simulink library "IO"  (R2024a)
settings: Solver=VariableStepAuto  StartTime=0.0  StopTime=10.0  RelTol=1e-3
values from neighbouring files (symbols this model uses):
  ADCBits = 12.0    [IO.sldd]
  DigitalPolarity : value not decoded    [IO.sldd]
  Vref = 5.0    [IO.sldd]
undefined symbols (not defined in the file or in its folder): Bridge, dt, enum2Raptor, H, raptor_xcp_function
libraries: Raptor_lib x118, Utilities x27, Cooling x1
(part 1 of 4)
settings Model: Creator=serga  LastModifiedBy=serga

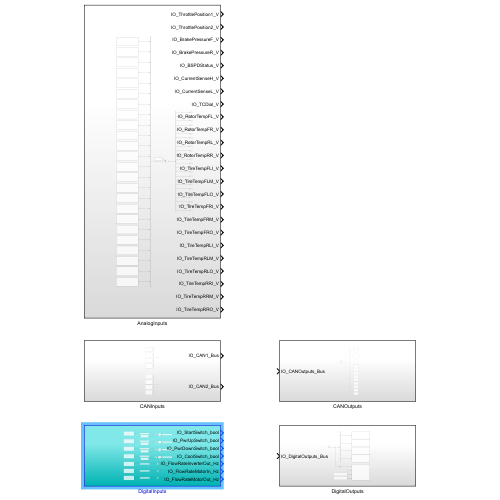
[thumbnail: Simulink's stored preview of the top-level diagram]
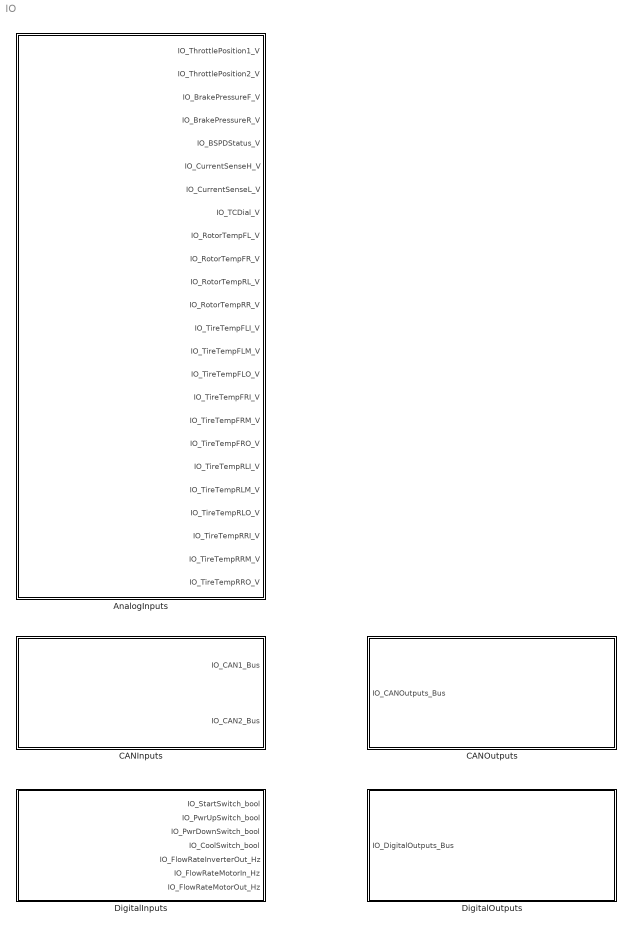
== system IO ==
  AnalogInputs : Subsystem
  CANInputs : Subsystem
  CANOutputs : Subsystem
  DigitalInputs : Subsystem
  DigitalOutputs : Subsystem

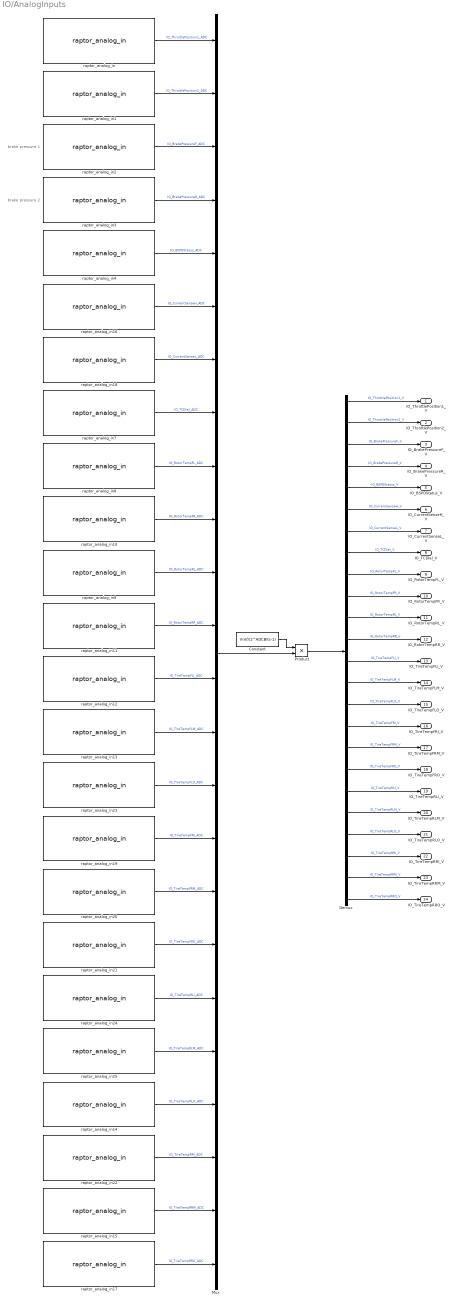
== system IO/AnalogInputs ==
  note: brake pressure 2
  note: brake pressure 1
  Constant : Constant  Value=Vref/(2^ADCBits-1)
  Demux : Demux  Outputs=24
  Mux : Mux  Inputs=24
  Product : Product
  raptor_analog_in : Raptor_lib/Input & Output/raptor_analog_in  resourceValues=INPUT2|INPUT3|INPUT4|INPUT5|INPUT6|INPUT7|INPUT8|INPUT9|INPUT10|INPUT11|INPUT12|INPUT13|INPUT14|INPUT15|INPUT16|INPUT17|INPUT18|INPUT19|INPUT20|INPUT21|INPUT22|INPUT23|INPUT24|INPUT25|INPUT26|INPUT27|INPUT28|INPUT29|INPUT30|INPUT31|INPUT32|(None)  resource=INPUT23  rangeValues=0 - 5 V  range=0 - 5 V  filterrateValues=[]  filterrate='RAPTOR MASK DEFAULT'  resolutionValues=[]  resolution=[]  pullUDValues=56.7k PD  pullUD=56.7k PD
      settings: SourceProductName=Raptor
  raptor_analog_in1 : Raptor_lib/Input & Output/raptor_analog_in  resourceValues=INPUT2|INPUT3|INPUT4|INPUT5|INPUT6|INPUT7|INPUT8|INPUT9|INPUT10|INPUT11|INPUT12|INPUT13|INPUT14|INPUT15|INPUT16|INPUT17|INPUT18|INPUT19|INPUT20|INPUT21|INPUT22|INPUT23|INPUT24|INPUT25|INPUT26|INPUT27|INPUT28|INPUT29|INPUT30|INPUT31|INPUT32|(None)  resource=INPUT24  rangeValues=0 - 5 V  range=0 - 5 V  filterrateValues=[]  filterrate='RAPTOR MASK DEFAULT'  resolutionValues=[]  resolution=[]  pullUDValues=56.7k PD  pullUD=56.7k PD
      settings: SourceProductName=Raptor
  raptor_analog_in10 : Raptor_lib/Input & Output/raptor_analog_in  resourceValues=INPUT2|INPUT3|INPUT4|INPUT5|INPUT6|INPUT7|INPUT8|INPUT9|INPUT10|INPUT11|INPUT12|INPUT13|INPUT14|INPUT15|INPUT16|INPUT17|INPUT18|INPUT19|INPUT20|INPUT21|INPUT22|INPUT23|INPUT24|INPUT25|INPUT26|INPUT27|INPUT28|INPUT29|INPUT30|INPUT31|INPUT32|(None)  resource=INPUT9  rangeValues=0 - 5 V  range=0 - 5 V  filterrateValues=[]  filterrate='RAPTOR MASK DEFAULT'  resolutionValues=[]  resolution=[]  pullUDValues=681k PU  pullUD=681k PU
      settings: SourceProductName=Raptor
  raptor_analog_in11 : Raptor_lib/Input & Output/raptor_analog_in  resourceValues=INPUT2|INPUT3|INPUT4|INPUT5|INPUT6|INPUT7|INPUT8|INPUT9|INPUT10|INPUT11|INPUT12|INPUT13|INPUT14|INPUT15|INPUT16|INPUT17|INPUT18|INPUT19|INPUT20|INPUT21|INPUT22|INPUT23|INPUT24|INPUT25|INPUT26|INPUT27|INPUT28|INPUT29|INPUT30|INPUT31|INPUT32|(None)  resource=INPUT10  rangeValues=0 - 5 V  range=0 - 5 V  filterrateValues=[]  filterrate='RAPTOR MASK DEFAULT'  resolutionValues=[]  resolution=[]  pullUDValues=681k PU  pullUD=681k PU
      settings: SourceProductName=Raptor
  raptor_analog_in12 : Raptor_lib/Input & Output/raptor_analog_in  resourceValues=INPUT2|INPUT3|INPUT4|INPUT5|INPUT6|INPUT7|INPUT8|INPUT9|INPUT10|INPUT11|INPUT12|INPUT13|INPUT14|INPUT15|INPUT16|INPUT17|INPUT18|INPUT19|INPUT20|INPUT21|INPUT22|INPUT23|INPUT24|INPUT25|INPUT26|INPUT27|INPUT28|INPUT29|INPUT30|INPUT31|INPUT32|(None)  resource=INPUT2  rangeValues=0 - 5 V  range=0 - 5 V  filterrateValues=[]  filterrate='RAPTOR MASK DEFAULT'  resolutionValues=[]  resolution=[]  pullUDValues=2.15k PU  pullUD=2.15k PU
      settings: SourceProductName=Raptor
  raptor_analog_in13 : Raptor_lib/Input & Output/raptor_analog_in  resourceValues=INPUT2|INPUT3|INPUT4|INPUT5|INPUT6|INPUT7|INPUT8|INPUT9|INPUT10|INPUT11|INPUT12|INPUT13|INPUT14|INPUT15|INPUT16|INPUT17|INPUT18|INPUT19|INPUT20|INPUT21|INPUT22|INPUT23|INPUT24|INPUT25|INPUT26|INPUT27|INPUT28|INPUT29|INPUT30|INPUT31|INPUT32|(None)  resource=INPUT3  rangeValues=0 - 5 V  range=0 - 5 V  filterrateValues=[]  filterrate='RAPTOR MASK DEFAULT'  resolutionValues=[]  resolution=[]  pullUDValues=2.15k PU  pullUD=2.15k PU
      settings: SourceProductName=Raptor
  raptor_analog_in14 : Raptor_lib/Input & Output/raptor_analog_in  resourceValues=INPUT2|INPUT3|INPUT4|INPUT5|INPUT6|INPUT7|INPUT8|INPUT9|INPUT10|INPUT11|INPUT12|INPUT13|INPUT14|INPUT15|INPUT16|INPUT17|INPUT18|INPUT19|INPUT20|INPUT21|INPUT22|INPUT23|INPUT24|INPUT25|INPUT26|INPUT27|INPUT28|INPUT29|INPUT30|INPUT31|INPUT32|(None)  resource=INPUT8  rangeValues=0 - 5 V  range=0 - 5 V  filterrateValues=[]  filterrate='RAPTOR MASK DEFAULT'  resolutionValues=[]  resolution=[]  pullUDValues=4.64k PU  pullUD=4.64k PU
      settings: SourceProductName=Raptor
  raptor_analog_in15 : Raptor_lib/Input & Output/raptor_analog_in  resourceValues=INPUT2|INPUT3|INPUT4|INPUT5|INPUT6|INPUT7|INPUT8|INPUT9|INPUT10|INPUT11|INPUT12|INPUT13|INPUT14|INPUT15|INPUT16|INPUT17|INPUT18|INPUT19|INPUT20|INPUT21|INPUT22|INPUT23|INPUT24|INPUT25|INPUT26|INPUT27|INPUT28|INPUT29|INPUT30|INPUT31|INPUT32|(None)  resource=INPUT11  rangeValues=0 - 5 V  range=0 - 5 V  filterrateValues=[]  filterrate='RAPTOR MASK DEFAULT'  resolutionValues=[]  resolution=[]  pullUDValues=681k PU  pullUD=681k PU
      settings: SourceProductName=Raptor
  raptor_analog_in16 : Raptor_lib/Input & Output/raptor_analog_in  resourceValues=INPUT2|INPUT3|INPUT4|INPUT5|INPUT6|INPUT7|INPUT8|INPUT9|INPUT10|INPUT11|INPUT12|INPUT13|INPUT14|INPUT15|INPUT16|INPUT17|INPUT18|INPUT19|INPUT20|INPUT21|INPUT22|INPUT23|INPUT24|INPUT25|INPUT26|INPUT27|INPUT28|INPUT29|INPUT30|INPUT31|INPUT32|(None)  resource=INPUT13  rangeValues=0 - 5 V  range=0 - 5 V  filterrateValues=[]  filterrate='RAPTOR MASK DEFAULT'  resolutionValues=[]  resolution=[]  pullUDValues=2.15k PU, 31.6k PD  pullUD=2.15k PU, 31.6k PD
      settings: SourceProductName=Raptor
  raptor_analog_in17 : Raptor_lib/Input & Output/raptor_analog_in  resourceValues=INPUT2|INPUT3|INPUT4|INPUT5|INPUT6|INPUT7|INPUT8|INPUT9|INPUT10|INPUT11|INPUT12|INPUT13|INPUT14|INPUT15|INPUT16|INPUT17|INPUT18|INPUT19|INPUT20|INPUT21|INPUT22|INPUT23|INPUT24|INPUT25|INPUT26|INPUT27|INPUT28|INPUT29|INPUT30|INPUT31|INPUT32|(None)  resource=INPUT14  rangeValues=0 - 5 V  range=0 - 5 V  filterrateValues=[]  filterrate='RAPTOR MASK DEFAULT'  resolutionValues=[]  resolution=[]  pullUDValues=681k PU  pullUD=681k PU
      settings: SourceProductName=Raptor
  raptor_analog_in18 : Raptor_lib/Input & Output/raptor_analog_in  resourceValues=INPUT2|INPUT3|INPUT4|INPUT5|INPUT6|INPUT7|INPUT8|INPUT9|INPUT10|INPUT11|INPUT12|INPUT13|INPUT14|INPUT15|INPUT16|INPUT17|INPUT18|INPUT19|INPUT20|INPUT21|INPUT22|INPUT23|INPUT24|INPUT25|INPUT26|INPUT27|INPUT28|INPUT29|INPUT30|INPUT31|INPUT32|(None)  resource=INPUT15  rangeValues=0 - 5 V  range=0 - 5 V  filterrateValues=[]  filterrate='RAPTOR MASK DEFAULT'  resolutionValues=[]  resolution=[]  pullUDValues=2.15k PU, 31.6k PD  pullUD=2.15k PU, 31.6k PD
      settings: SourceProductName=Raptor
  raptor_analog_in19 : Raptor_lib/Input & Output/raptor_analog_in  resourceValues=INPUT2|INPUT3|INPUT4|INPUT5|INPUT6|INPUT7|INPUT8|INPUT9|INPUT10|INPUT11|INPUT12|INPUT13|INPUT14|INPUT15|INPUT16|INPUT17|INPUT18|INPUT19|INPUT20|INPUT21|INPUT22|INPUT23|INPUT24|INPUT25|INPUT26|INPUT27|INPUT28|INPUT29|INPUT30|INPUT31|INPUT32|(None)  resource=INPUT16  rangeValues=0 - 5 V  range=0 - 5 V  filterrateValues=[]  filterrate='RAPTOR MASK DEFAULT'  resolutionValues=[]  resolution=[]  pullUDValues=4.64k PU  pullUD=4.64k PU
      settings: SourceProductName=Raptor
  raptor_analog_in2 : Raptor_lib/Input & Output/raptor_analog_in  resourceValues=INPUT2|INPUT3|INPUT4|INPUT5|INPUT6|INPUT7|INPUT8|INPUT9|INPUT10|INPUT11|INPUT12|INPUT13|INPUT14|INPUT15|INPUT16|INPUT17|INPUT18|INPUT19|INPUT20|INPUT21|INPUT22|INPUT23|INPUT24|INPUT25|INPUT26|INPUT27|INPUT28|INPUT29|INPUT30|INPUT31|INPUT32|(None)  resource=INPUT4  rangeValues=0 - 5 V  range=0 - 5 V  filterrateValues=[]  filterrate='RAPTOR MASK DEFAULT'  resolutionValues=[]  resolution=[]  pullUDValues=422k PD  pullUD=422k PD
      settings: SourceProductName=Raptor
  raptor_analog_in20 : Raptor_lib/Input & Output/raptor_analog_in  resourceValues=INPUT2|INPUT3|INPUT4|INPUT5|INPUT6|INPUT7|INPUT8|INPUT9|INPUT10|INPUT11|INPUT12|INPUT13|INPUT14|INPUT15|INPUT16|INPUT17|INPUT18|INPUT19|INPUT20|INPUT21|INPUT22|INPUT23|INPUT24|INPUT25|INPUT26|INPUT27|INPUT28|INPUT29|INPUT30|INPUT31|INPUT32|(None)  resource=INPUT19  rangeValues=0 - 5 V  range=0 - 5 V  filterrateValues=[]  filterrate='RAPTOR MASK DEFAULT'  resolutionValues=[]  resolution=[]  pullUDValues=2.15k PU  pullUD=2.15k PU
      settings: SourceProductName=Raptor
  raptor_analog_in21 : Raptor_lib/Input & Output/raptor_analog_in  resourceValues=INPUT2|INPUT3|INPUT4|INPUT5|INPUT6|INPUT7|INPUT8|INPUT9|INPUT10|INPUT11|INPUT12|INPUT13|INPUT14|INPUT15|INPUT16|INPUT17|INPUT18|INPUT19|INPUT20|INPUT21|INPUT22|INPUT23|INPUT24|INPUT25|INPUT26|INPUT27|INPUT28|INPUT29|INPUT30|INPUT31|INPUT32|(None)  resource=INPUT21  rangeValues=0 - 5 V  range=0 - 5 V  filterrateValues=[]  filterrate='RAPTOR MASK DEFAULT'  resolutionValues=[]  resolution=[]  pullUDValues=2.15k PU  pullUD=2.15k PU
      settings: SourceProductName=Raptor
  raptor_analog_in22 : Raptor_lib/Input & Output/raptor_analog_in  resourceValues=INPUT2|INPUT3|INPUT4|INPUT5|INPUT6|INPUT7|INPUT8|INPUT9|INPUT10|INPUT11|INPUT12|INPUT13|INPUT14|INPUT15|INPUT16|INPUT17|INPUT18|INPUT19|INPUT20|INPUT21|INPUT22|INPUT23|INPUT24|INPUT25|INPUT26|INPUT27|INPUT28|INPUT29|INPUT30|INPUT31|INPUT32|(None)  resource=INPUT22  rangeValues=0 - 5 V  range=0 - 5 V  filterrateValues=[]  filterrate='RAPTOR MASK DEFAULT'  resolutionValues=[]  resolution=[]  pullUDValues=2.15k PU  pullUD=2.15k PU
      settings: SourceProductName=Raptor
  raptor_analog_in23 : Raptor_lib/Input & Output/raptor_analog_in  resourceValues=INPUT2|INPUT3|INPUT4|INPUT5|INPUT6|INPUT7|INPUT8|INPUT9|INPUT10|INPUT11|INPUT12|INPUT13|INPUT14|INPUT15|INPUT16|INPUT17|INPUT18|INPUT19|INPUT20|INPUT21|INPUT22|INPUT23|INPUT24|INPUT25|INPUT26|INPUT27|INPUT28|INPUT29|INPUT30|INPUT31|INPUT32|(None)  resource=INPUT25  rangeValues=0 - 5 V  range=0 - 5 V  filterrateValues=[]  filterrate='RAPTOR MASK DEFAULT'  resolutionValues=[]  resolution=[]  pullUDValues=2.15k PU  pullUD=2.15k PU
      settings: SourceProductName=Raptor
  raptor_analog_in24 : Raptor_lib/Input & Output/raptor_analog_in  resourceValues=INPUT2|INPUT3|INPUT4|INPUT5|INPUT6|INPUT7|INPUT8|INPUT9|INPUT10|INPUT11|INPUT12|INPUT13|INPUT14|INPUT15|INPUT16|INPUT17|INPUT18|INPUT19|INPUT20|INPUT21|INPUT22|INPUT23|INPUT24|INPUT25|INPUT26|INPUT27|INPUT28|INPUT29|INPUT30|INPUT31|INPUT32|(None)  resource=INPUT26  rangeValues=0 - 5 V  range=0 - 5 V  filterrateValues=[]  filterrate='RAPTOR MASK DEFAULT'  resolutionValues=[]  resolution=[]  pullUDValues=681k PU  pullUD=681k PU
      settings: SourceProductName=Raptor
  raptor_analog_in25 : Raptor_lib/Input & Output/raptor_analog_in  resourceValues=INPUT2|INPUT3|INPUT4|INPUT5|INPUT6|INPUT7|INPUT8|INPUT9|INPUT10|INPUT11|INPUT12|INPUT13|INPUT14|INPUT15|INPUT16|INPUT17|INPUT18|INPUT19|INPUT20|INPUT21|INPUT22|INPUT23|INPUT24|INPUT25|INPUT26|INPUT27|INPUT28|INPUT29|INPUT30|INPUT31|INPUT32|(None)  resource=INPUT28  rangeValues=0 - 5 V  range=0 - 5 V  filterrateValues=[]  filterrate='RAPTOR MASK DEFAULT'  resolutionValues=[]  resolution=[]  pullUDValues=2.15k PU  pullUD=2.15k PU
      settings: SourceProductName=Raptor
  raptor_analog_in3 : Raptor_lib/Input & Output/raptor_analog_in  resourceValues=INPUT2|INPUT3|INPUT4|INPUT5|INPUT6|INPUT7|INPUT8|INPUT9|INPUT10|INPUT11|INPUT12|INPUT13|INPUT14|INPUT15|INPUT16|INPUT17|INPUT18|INPUT19|INPUT20|INPUT21|INPUT22|INPUT23|INPUT24|INPUT25|INPUT26|INPUT27|INPUT28|INPUT29|INPUT30|INPUT31|INPUT32|(None)  resource=INPUT12  rangeValues=0 - 5 V  range=0 - 5 V  filterrateValues=[]  filterrate='RAPTOR MASK DEFAULT'  resolutionValues=[]  resolution=[]  pullUDValues=422k PD  pullUD=422k PD
      settings: SourceProductName=Raptor
  raptor_analog_in4 : Raptor_lib/Input & Output/raptor_analog_in  resourceValues=INPUT2|INPUT3|INPUT4|INPUT5|INPUT6|INPUT7|INPUT8|INPUT9|INPUT10|INPUT11|INPUT12|INPUT13|INPUT14|INPUT15|INPUT16|INPUT17|INPUT18|INPUT19|INPUT20|INPUT21|INPUT22|INPUT23|INPUT24|INPUT25|INPUT26|INPUT27|INPUT28|INPUT29|INPUT30|INPUT31|INPUT32|(None)  resource=INPUT18  rangeValues=0 - 5 V  range=0 - 5 V  filterrateValues=[]  filterrate='RAPTOR MASK DEFAULT'  resolutionValues=[]  resolution=[]  pullUDValues=422k PD  pullUD=422k PD
      settings: SourceProductName=Raptor
  raptor_analog_in7 : Raptor_lib/Input & Output/raptor_analog_in  resourceValues=INPUT2|INPUT3|INPUT4|INPUT5|INPUT6|INPUT7|INPUT8|INPUT9|INPUT10|INPUT11|INPUT12|INPUT13|INPUT14|INPUT15|INPUT16|INPUT17|INPUT18|INPUT19|INPUT20|INPUT21|INPUT22|INPUT23|INPUT24|INPUT25|INPUT26|INPUT27|INPUT28|INPUT29|INPUT30|INPUT31|INPUT32|(None)  resource=INPUT29  rangeValues=0 - 5 V  range=0 - 5 V  filterrateValues=[]  filterrate='RAPTOR MASK DEFAULT'  resolutionValues=[]  resolution=[]  pullUDValues=215k PD  pullUD=215k PD
      settings: SourceProductName=Raptor
  raptor_analog_in8 : Raptor_lib/Input & Output/raptor_analog_in  resourceValues=INPUT2|INPUT3|INPUT4|INPUT5|INPUT6|INPUT7|INPUT8|INPUT9|INPUT10|INPUT11|INPUT12|INPUT13|INPUT14|INPUT15|INPUT16|INPUT17|INPUT18|INPUT19|INPUT20|INPUT21|INPUT22|INPUT23|INPUT24|INPUT25|INPUT26|INPUT27|INPUT28|INPUT29|INPUT30|INPUT31|INPUT32|(None)  resource=INPUT6  rangeValues=0 - 5 V  range=0 - 5 V  filterrateValues=[]  filterrate='RAPTOR MASK DEFAULT'  resolutionValues=[]  resolution=[]  pullUDValues=681k PU  pullUD=681k PU
      settings: SourceProductName=Raptor
  raptor_analog_in9 : Raptor_lib/Input & Output/raptor_analog_in  resourceValues=INPUT2|INPUT3|INPUT4|INPUT5|INPUT6|INPUT7|INPUT8|INPUT9|INPUT10|INPUT11|INPUT12|INPUT13|INPUT14|INPUT15|INPUT16|INPUT17|INPUT18|INPUT19|INPUT20|INPUT21|INPUT22|INPUT23|INPUT24|INPUT25|INPUT26|INPUT27|INPUT28|INPUT29|INPUT30|INPUT31|INPUT32|(None)  resource=INPUT7  rangeValues=0 - 5 V  range=0 - 5 V  filterrateValues=[]  filterrate='RAPTOR MASK DEFAULT'  resolutionValues=[]  resolution=[]  pullUDValues=681k PU  pullUD=681k PU
      settings: SourceProductName=Raptor
  IO_ThrottlePosition1_V : Outport
  IO_ThrottlePosition2_V : Outport  Port=2
  IO_BrakePressureF_V : Outport  Port=3
  IO_BrakePressureR_V : Outport  Port=4
  IO_BSPDStatus_V : Outport  Port=5
  IO_CurrentSenseH_V : Outport  Port=6
  IO_CurrentSenseL_V : Outport  Port=7
  IO_TCDial_V : Outport  Port=8
  IO_RotorTempFL_V : Outport  Port=9
  IO_RotorTempFR_V : Outport  Port=10
  IO_RotorTempRL_V : Outport  Port=11
  IO_RotorTempRR_V : Outport  Port=12
  IO_TireTempFLI_V : Outport  Port=13
  IO_TireTempFLM_V : Outport  Port=14
  IO_TireTempFLO_V : Outport  Port=15
  IO_TireTempFRI_V : Outport  Port=16
  IO_TireTempFRM_V : Outport  Port=17
  IO_TireTempFRO_V : Outport  Port=18
  IO_TireTempRLI_V : Outport  Port=19
  IO_TireTempRLM_V : Outport  Port=20
  IO_TireTempRLO_V : Outport  Port=21
  IO_TireTempRRI_V : Outport  Port=22
  IO_TireTempRRM_V : Outport  Port=23
  IO_TireTempRRO_V : Outport  Port=24
  wires:
  Demux/24 -> IO_TireTempRRO_V/1  "IO_TireTempRRO_V"
  Demux/23 -> IO_TireTempRRM_V/1  "IO_TireTempRRM_V"
  Demux/22 -> IO_TireTempRRI_V/1  "IO_TireTempRRI_V"
  Demux/21 -> IO_TireTempRLO_V/1  "IO_TireTempRLO_V"
  Demux/20 -> IO_TireTempRLM_V/1  "IO_TireTempRLM_V"
  Demux/19 -> IO_TireTempRLI_V/1  "IO_TireTempRLI_V"
  Demux/18 -> IO_TireTempFRO_V/1  "IO_TireTempFRO_V"
  Demux/17 -> IO_TireTempFRM_V/1  "IO_TireTempFRM_V"
  Demux/16 -> IO_TireTempFRI_V/1  "IO_TireTempFRI_V"
  Demux/15 -> IO_TireTempFLO_V/1  "IO_TireTempFLO_V"
  Demux/14 -> IO_TireTempFLM_V/1  "IO_TireTempFLM_V"
  Demux/13 -> IO_TireTempFLI_V/1  "IO_TireTempFLI_V"
  raptor_analog_in25/1 -> Mux/20  "IO_TireTempRLM_ADC"
  raptor_analog_in24/1 -> Mux/19  "IO_TireTempRLI_ADC"
  raptor_analog_in23/1 -> Mux/15  "IO_TireTempFLO_ADC"
  raptor_analog_in22/1 -> Mux/22  "IO_TireTempRRI_ADC"
  raptor_analog_in21/1 -> Mux/18  "IO_TireTempFRO_ADC"
  raptor_analog_in20/1 -> Mux/17  "IO_TireTempFRM_ADC"
  raptor_analog_in19/1 -> Mux/16  "IO_TireTempFRI_ADC"
  raptor_analog_in18/1 -> Mux/7  "IO_CurrentSenseL_ADC"
  raptor_analog_in17/1 -> Mux/24  "IO_TireTempRRO_ADC"
  raptor_analog_in16/1 -> Mux/6  "IO_CurrentSenseH_ADC"
  raptor_analog_in15/1 -> Mux/23  "IO_TireTempRRM_ADC"
  raptor_analog_in14/1 -> Mux/21  "IO_TireTempRLO_ADC"
  raptor_analog_in13/1 -> Mux/14  "IO_TireTempFLM_ADC"
  raptor_analog_in12/1 -> Mux/13  "IO_TireTempFLI_ADC"
  Demux/12 -> IO_RotorTempRR_V/1  "IO_RotorTempRR_V"
  Demux/11 -> IO_RotorTempRL_V/1  "IO_RotorTempRL_V"
  Demux/10 -> IO_RotorTempFR_V/1  "IO_RotorTempFR_V"
  Demux/9 -> IO_RotorTempFL_V/1  "IO_RotorTempFL_V"
  Demux/8 -> IO_TCDial_V/1  "IO_TCDial_V"
  Demux/7 -> IO_CurrentSenseL_V/1  "IO_CurrentSenseL_V"
  Demux/6 -> IO_CurrentSenseH_V/1  "IO_CurrentSenseH_V"
  Demux/5 -> IO_BSPDStatus_V/1  "IO_BSPDStatus_V"
  raptor_analog_in11/1 -> Mux/12  "IO_RotorTempRR_ADC"
  raptor_analog_in10/1 -> Mux/10  "IO_RotorTempFR_ADC"
  raptor_analog_in9/1 -> Mux/11  "IO_RotorTempRL_ADC"
  raptor_analog_in8/1 -> Mux/9  "IO_RotorTempFL_ADC"
  raptor_analog_in7/1 -> Mux/8  "IO_TCDial_ADC"
  raptor_analog_in4/1 -> Mux/5  "IO_BSPDStatus_ADC"
  Demux/4 -> IO_BrakePressureR_V/1  "IO_BrakePressureR_V"
  Demux/3 -> IO_BrakePressureF_V/1  "IO_BrakePressureF_V"
  raptor_analog_in3/1 -> Mux/4  "IO_BrakePressureR_ADC"
  raptor_analog_in2/1 -> Mux/3  "IO_BrakePressureF_ADC"
  Constant/1 -> Product/1
  Mux/1 -> Product/2
  Product/1 -> Demux/1
  raptor_analog_in/1 -> Mux/1  "IO_ThrottlePosition1_ADC"
  Demux/1 -> IO_ThrottlePosition1_V/1  "IO_ThrottlePosition1_V"
  raptor_analog_in1/1 -> Mux/2  "IO_ThrottlePosition2_ADC"
  Demux/2 -> IO_ThrottlePosition2_V/1  "IO_ThrottlePosition2_V"

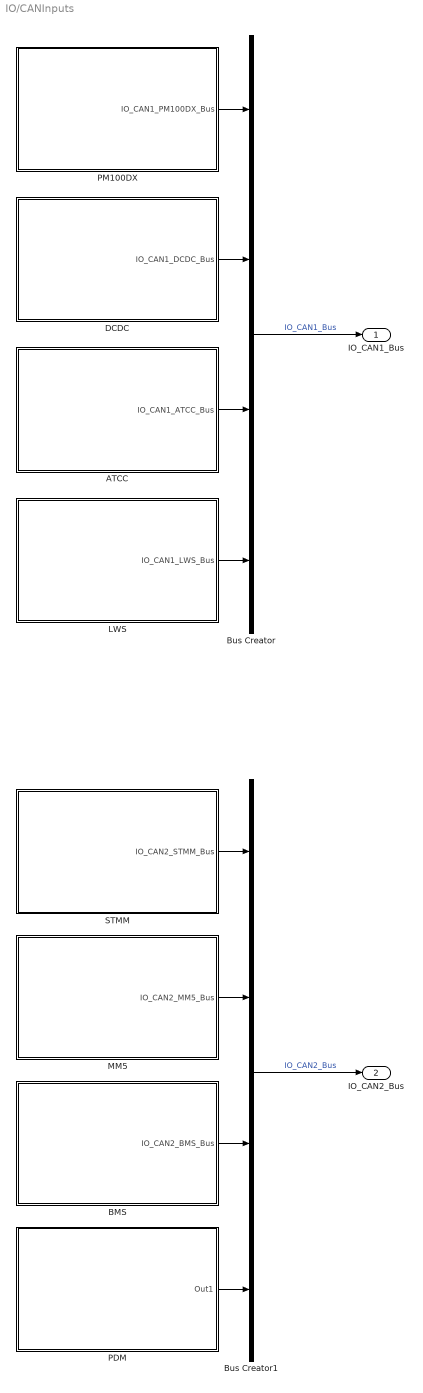
== system IO/CANInputs ==
  ATCC : Subsystem
  BMS : Subsystem
  Bus Creator : BusCreator  Inputs=4
  Bus Creator1 : BusCreator  Inputs=4
  DCDC : Subsystem
  LWS : Subsystem
  MM5 : Subsystem
  PDM : Subsystem
  PM100DX : Subsystem
  STMM : Subsystem
  IO_CAN1_Bus : Outport
  IO_CAN2_Bus : Outport  Port=2
  wires:
  PDM/1(Out1) -> Bus Creator1/4
  BMS/1(IO_CAN2_BMS_Bus) -> Bus Creator1/3
  LWS/1(IO_CAN1_LWS_Bus) -> Bus Creator/4
  ATCC/1(IO_CAN1_ATCC_Bus) -> Bus Creator/3
  MM5/1(IO_CAN2_MM5_Bus) -> Bus Creator1/2
  STMM/1(IO_CAN2_STMM_Bus) -> Bus Creator1/1
  DCDC/1(IO_CAN1_DCDC_Bus) -> Bus Creator/2
  Bus Creator1/1 -> IO_CAN2_Bus/1  "IO_CAN2_Bus"
  Bus Creator/1 -> IO_CAN1_Bus/1  "IO_CAN1_Bus"
  PM100DX/1(IO_CAN1_PM100DX_Bus) -> Bus Creator/1

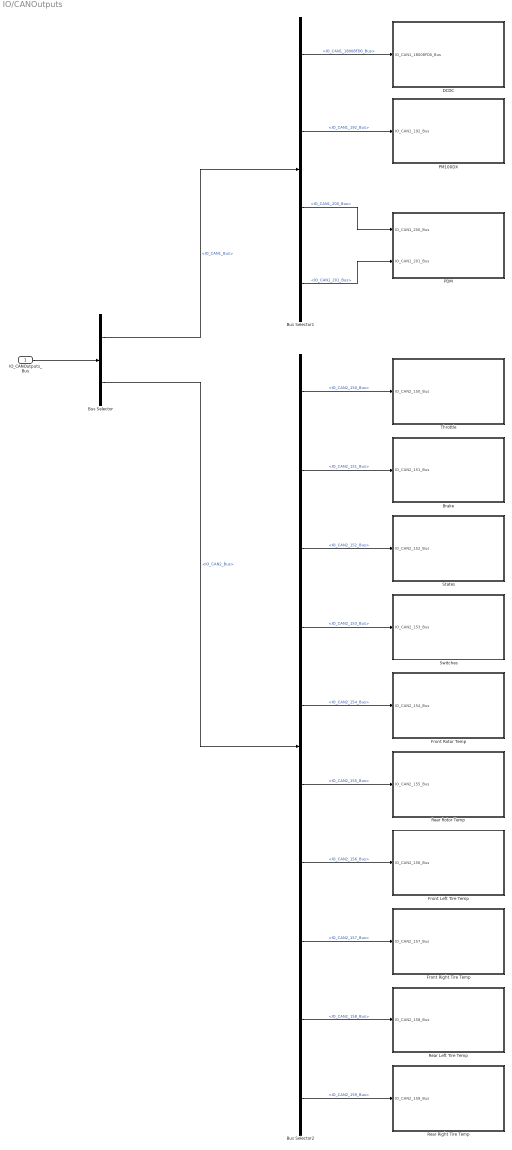
== system IO/CANOutputs ==
  IO_CANOutputs_Bus : Inport
  Brake : Subsystem
  Bus Selector : BusSelector  OutputSignals=IO_CAN1_Bus,IO_CAN2_Bus
  Bus Selector1 : BusSelector  OutputSignals=IO_CAN1_18008FD0_Bus,IO_CAN1_192_Bus,IO_CAN1_200_Bus,IO_CAN1_201_Bus
  Bus Selector2 : BusSelector  OutputSignals=IO_CAN2_150_Bus,IO_CAN2_151_Bus,IO_CAN2_152_Bus,IO_CAN2_153_Bus,IO_CAN2_154_Bus,IO_CAN2_155_Bus,IO_CAN2_156_Bus,IO_CAN2_157_Bus,IO_CAN2_158_Bus,IO_CAN2_159_Bus
  DCDC : Subsystem
  Front Left Tire Temp : Subsystem
  Front Right Tire Temp : Subsystem
  Front Rotor Temp : Subsystem
  PDM : Subsystem
  PM100DX : Subsystem
  Rear Left Tire Temp : Subsystem
  Rear Right Tire Temp : Subsystem
  Rear Rotor Temp : Subsystem
  States : Subsystem
  Switches : Subsystem
  Throttle : Subsystem
  wires:
  Bus Selector2/10 -> Rear Right Tire Temp/1(IO_CAN2_159_Bus)  "<IO_CAN2_159_Bus>"
  Bus Selector2/9 -> Rear Left Tire Temp/1(IO_CAN2_158_Bus)  "<IO_CAN2_158_Bus>"
  Bus Selector2/8 -> Front Right Tire Temp/1(IO_CAN2_157_Bus)  "<IO_CAN2_157_Bus>"
  Bus Selector2/7 -> Front Left Tire Temp/1(IO_CAN2_156_Bus)  "<IO_CAN2_156_Bus>"
  Bus Selector2/6 -> Rear Rotor Temp/1(IO_CAN2_155_Bus)  "<IO_CAN2_155_Bus>"
  Bus Selector2/5 -> Front Rotor Temp/1(IO_CAN2_154_Bus)  "<IO_CAN2_154_Bus>"
  Bus Selector1/4 -> PDM/2(IO_CAN1_201_Bus)  "<IO_CAN1_201_Bus>"
  Bus Selector2/4 -> Switches/1(IO_CAN2_153_Bus)  "<IO_CAN2_153_Bus>"
  Bus Selector2/3 -> States/1(IO_CAN2_152_Bus)  "<IO_CAN2_152_Bus>"
  Bus Selector2/2 -> Brake/1(IO_CAN2_151_Bus)  "<IO_CAN2_151_Bus>"
  Bus Selector2/1 -> Throttle/1(IO_CAN2_150_Bus)  "<IO_CAN2_150_Bus>"
  Bus Selector/2 -> Bus Selector2/1  "<IO_CAN2_Bus>"
  Bus Selector1/3 -> PDM/1(IO_CAN1_200_Bus)  "<IO_CAN1_200_Bus>"
  Bus Selector1/2 -> PM100DX/1(IO_CAN1_192_Bus)  "<IO_CAN1_192_Bus>"
  Bus Selector1/1 -> DCDC/1(IO_CAN1_18008FD0_Bus)  "<IO_CAN1_18008FD0_Bus>"
  Bus Selector/1 -> Bus Selector1/1  "<IO_CAN1_Bus>"
  IO_CANOutputs_Bus/1 -> Bus Selector/1

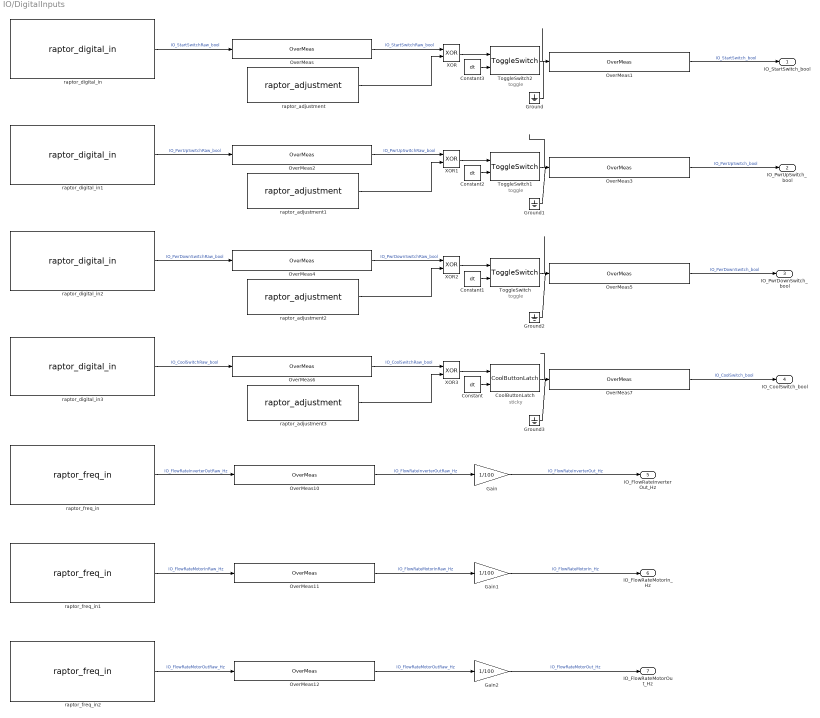
== system IO/DigitalInputs ==
  note: toggle
  note: sticky
  note: toggle
  note: toggle
  Constant{,1..3} (4 alike) : Constant  Value=dt
  CoolButtonLatch : Cooling/CoolButtonLatch  SystemSampleTime=-1  VariantActivationTime=update diagram  AllowFlexibleInterface=on  Latency=0  AutoFrameSizeCalculation=off
  Gain : Gain  Gain=1/100  OutDataTypeStr=single
  Gain1 : Gain  Gain=1/100  OutDataTypeStr=single
  Gain2 : Gain  Gain=1/100  OutDataTypeStr=single
  Ground{,1..3} (4 alike) : Ground
  OverMeas : Utilities/OverMeas  sigName='IO_StartSwitchRaw_bool'  minimum=0  maximum=1
  OverMeas1 : Utilities/OverMeas  sigName='IO_StartSwitch_bool'  minimum=0  maximum=1
  OverMeas10 : Utilities/OverMeas  sigName='IO_FlowRateInverterOutRaw_Hz'  minimum=-inf  maximum=inf
  OverMeas11 : Utilities/OverMeas  sigName='IO_FlowRateMotorInRaw_Hz'  minimum=-inf  maximum=inf
  OverMeas12 : Utilities/OverMeas  sigName='IO_FlowRateMotorOutRaw_Hz'  minimum=-inf  maximum=inf
  OverMeas2 : Utilities/OverMeas  sigName='IO_PwrUpSwitchRaw_bool'  minimum=0  maximum=1
  OverMeas3 : Utilities/OverMeas  sigName='IO_PwrUpSwitch_bool'  minimum=0  maximum=1
  OverMeas4 : Utilities/OverMeas  sigName='IO_PwrDownSwitchRaw_bool'  minimum=0  maximum=1
  OverMeas5 : Utilities/OverMeas  sigName='IO_PwrDownSwitch_bool'  minimum=0  maximum=1
  OverMeas6 : Utilities/OverMeas  sigName='IO_CoolSwitchRaw_bool'  minimum=0  maximum=1
  OverMeas7 : Utilities/OverMeas  sigName='IO_CoolSwitch_bool'  minimum=0  maximum=1
  ToggleSwitch : Utilities/ToggleSwitch  SystemSampleTime=-1  VariantActivationTime=update diagram  AllowFlexibleInterface=on  Latency=0  AutoFrameSizeCalculation=off
  ToggleSwitch1 : Utilities/ToggleSwitch  SystemSampleTime=-1  VariantActivationTime=update diagram  AllowFlexibleInterface=on  Latency=0  AutoFrameSizeCalculation=off
  ToggleSwitch2 : Utilities/ToggleSwitch  SystemSampleTime=-1  VariantActivationTime=update diagram  AllowFlexibleInterface=on  Latency=0  AutoFrameSizeCalculation=off
  XOR{,1..3} (4 alike) : Logic  Operator=XOR  AllPortsSameDT=off  OutDataTypeStr=boolean
  raptor_adjustment : Raptor_lib/Data Storage/raptor_adjustment  paramName='IO_StartSwitchPolarity_bool'  nameSource=Parameter  initValue=DigitalPolarity.ActiveHigh  dataType=uint8  storage=Calibration  calDispType=Enumeration  calEnum=enum2Raptor(DigitalPolarity.ActiveHigh)  calGain=1.0  calOffset=0.0  calMax=inf  calMin=-inf  calFormat='-1'  calUnit=''  calHelp=''  calAccess=1  calFunction=raptor_xcp_function(gcb)  calDispHeaders=off  calColHeaders={'Col1' 'Col2' 'Col3'}  calRowHeaders={'Row1' 'Row2' 'Row3'}
      settings: SourceProductName=Raptor
  raptor_adjustment1 : Raptor_lib/Data Storage/raptor_adjustment  paramName='IO_PwrUpSwitchPolarity_bool'  nameSource=Parameter  initValue=DigitalPolarity.ActiveHigh  dataType=uint8  storage=Calibration  calDispType=Enumeration  calEnum=enum2Raptor(DigitalPolarity.ActiveHigh)  calGain=1.0  calOffset=0.0  calMax=inf  calMin=-inf  calFormat='-1'  calUnit=''  calHelp=''  calAccess=1  calFunction=raptor_xcp_function(gcb)  calDispHeaders=off  calColHeaders={'Col1' 'Col2' 'Col3'}  calRowHeaders={'Row1' 'Row2' 'Row3'}
      settings: SourceProductName=Raptor
  raptor_adjustment2 : Raptor_lib/Data Storage/raptor_adjustment  paramName='IO_PwrDownSwitchPolarity_bool'  nameSource=Parameter  initValue=DigitalPolarity.ActiveHigh  dataType=uint8  storage=Calibration  calDispType=Enumeration  calEnum=enum2Raptor(DigitalPolarity.ActiveHigh)  calGain=1.0  calOffset=0.0  calMax=inf  calMin=-inf  calFormat='-1'  calUnit=''  calHelp=''  calAccess=1  calFunction=raptor_xcp_function(gcb)  calDispHeaders=off  calColHeaders={'Col1' 'Col2' 'Col3'}  calRowHeaders={'Row1' 'Row2' 'Row3'}
      settings: SourceProductName=Raptor
  raptor_adjustment3 : Raptor_lib/Data Storage/raptor_adjustment  paramName='IO_CoolSwitchPolarity_bool'  nameSource=Parameter  initValue=DigitalPolarity.ActiveHigh  dataType=uint8  storage=Calibration  calDispType=Enumeration  calEnum=enum2Raptor(DigitalPolarity.ActiveHigh)  calGain=1.0  calOffset=0.0  calMax=inf  calMin=-inf  calFormat='-1'  calUnit=''  calHelp=''  calAccess=1  calFunction=raptor_xcp_function(gcb)  calDispHeaders=off  calColHeaders={'Col1' 'Col2' 'Col3'}  calRowHeaders={'Row1' 'Row2' 'Row3'}
      settings: SourceProductName=Raptor
  raptor_digital_in : Raptor_lib/Input & Output/raptor_digital_in  resourceValues=WAKE_INPUT1|INPUT33|INPUT34|INPUT35|INPUT36|INPUT37|INPUT38|INPUT39|INPUT40|(None)  resource=INPUT35  pullUDValues=1.3k PD  pullUD=1.3k PD  upperThres='RAPTOR MASK DEFAULT'  lowerThres='RAPTOR MASK DEFAULT'
      settings: SourceProductName=Raptor
  raptor_digital_in1 : Raptor_lib/Input & Output/raptor_digital_in  resourceValues=WAKE_INPUT1|INPUT33|INPUT34|INPUT35|INPUT36|INPUT37|INPUT38|INPUT39|INPUT40|(None)  resource=INPUT37  pullUDValues=1.3k PU  pullUD=1.3k PU  upperThres='RAPTOR MASK DEFAULT'  lowerThres='RAPTOR MASK DEFAULT'
      settings: SourceProductName=Raptor
  raptor_digital_in2 : Raptor_lib/Input & Output/raptor_digital_in  resourceValues=WAKE_INPUT1|INPUT33|INPUT34|INPUT35|INPUT36|INPUT37|INPUT38|INPUT39|INPUT40|(None)  resource=INPUT39  pullUDValues=1.3k PU  pullUD=1.3k PU  upperThres='RAPTOR MASK DEFAULT'  lowerThres='RAPTOR MASK DEFAULT'
      settings: SourceProductName=Raptor
  raptor_digital_in3 : Raptor_lib/Input & Output/raptor_digital_in  resourceValues=WAKE_INPUT1|INPUT33|INPUT34|INPUT35|INPUT36|INPUT37|INPUT38|INPUT39|INPUT40|(None)  resource=INPUT40  pullUDValues=1.3k PU  pullUD=1.3k PU  upperThres='RAPTOR MASK DEFAULT'  lowerThres='RAPTOR MASK DEFAULT'
      settings: SourceProductName=Raptor
  raptor_freq_in : Raptor_lib/Input & Output/raptor_freq_in  minFreq=1  resourceValues=INPUT41|INPUT42|INPUT43|INPUT44|INPUT45|(None)  resource=INPUT43  pullUDValues=[]  pullUD=[]  interfaceValues=[]  interface=[]  dcEdgeValues=Rising | Falling  dcEdge=Rising  hasDuty=off  hasEdgeCount=off
      settings: SourceProductName=Raptor
  raptor_freq_in1 : Raptor_lib/Input & Output/raptor_freq_in  minFreq=1  resourceValues=INPUT41|INPUT42|INPUT43|INPUT44|INPUT45|(None)  resource=INPUT41  pullUDValues=[]  pullUD=[]  interfaceValues=[]  interface=[]  dcEdgeValues=Rising | Falling  dcEdge=Rising  hasDuty=off  hasEdgeCount=off
      settings: SourceProductName=Raptor
  raptor_freq_in2 : Raptor_lib/Input & Output/raptor_freq_in  minFreq=1  resourceValues=INPUT41|INPUT42|INPUT43|INPUT44|INPUT45|(None)  resource=INPUT44  pullUDValues=[]  pullUD=[]  interfaceValues=[]  interface=[]  dcEdgeValues=Rising | Falling  dcEdge=Rising  hasDuty=off  hasEdgeCount=off
      settings: SourceProductName=Raptor
  IO_StartSwitch_bool : Outport
  IO_PwrUpSwitch_bool : Outport  Port=2
  IO_PwrDownSwitch_bool : Outport  Port=3
  IO_CoolSwitch_bool : Outport  Port=4
  IO_FlowRateInverterOut_Hz : Outport  Port=5
  IO_FlowRateMotorIn_Hz : Outport  Port=6
  IO_FlowRateMotorOut_Hz : Outport  Port=7
  wires:
  Gain2/1 -> IO_FlowRateMotorOut_Hz/1  "IO_FlowRateMotorOut_Hz"
  OverMeas12/1 -> Gain2/1  "IO_FlowRateMotorOutRaw_Hz"
  Gain1/1 -> IO_FlowRateMotorIn_Hz/1  "IO_FlowRateMotorIn_Hz"
  OverMeas11/1 -> Gain1/1  "IO_FlowRateMotorInRaw_Hz"
  raptor_freq_in2/1 -> OverMeas12/1  "IO_FlowRateMotorOutRaw_Hz"
  raptor_freq_in1/1 -> OverMeas11/1  "IO_FlowRateMotorInRaw_Hz"
  XOR3/1 -> CoolButtonLatch/1
  XOR2/1 -> ToggleSwitch/1
  XOR1/1 -> ToggleSwitch1/1
  OverMeas10/1 -> Gain/1  "IO_FlowRateInverterOutRaw_Hz"
  Gain/1 -> IO_FlowRateInverterOut_Hz/1  "IO_FlowRateInverterOut_Hz"
  raptor_freq_in/1 -> OverMeas10/1  "IO_FlowRateInverterOutRaw_Hz"
  OverMeas7/1 -> IO_CoolSwitch_bool/1  "IO_CoolSwitch_bool"
  raptor_adjustment3/1 -> XOR3/2
  OverMeas6/1 -> XOR3/1  "IO_CoolSwitchRaw_bool"
  OverMeas5/1 -> IO_PwrDownSwitch_bool/1  "IO_PwrDownSwitch_bool"
  OverMeas4/1 -> XOR2/1  "IO_PwrDownSwitchRaw_bool"
  raptor_adjustment2/1 -> XOR2/2
  raptor_adjustment1/1 -> XOR1/2
  OverMeas3/1 -> IO_PwrUpSwitch_bool/1  "IO_PwrUpSwitch_bool"
  OverMeas2/1 -> XOR1/1  "IO_PwrUpSwitchRaw_bool"
  OverMeas1/1 -> IO_StartSwitch_bool/1  "IO_StartSwitch_bool"
  OverMeas/1 -> XOR/1  "IO_StartSwitchRaw_bool"
  raptor_adjustment/1 -> XOR/2
  raptor_digital_in3/1 -> OverMeas6/1  "IO_CoolSwitchRaw_bool"
  raptor_digital_in2/1 -> OverMeas4/1  "IO_PwrDownSwitchRaw_bool"
  raptor_digital_in1/1 -> OverMeas2/1  "IO_PwrUpSwitchRaw_bool"
  raptor_digital_in/1 -> OverMeas/1  "IO_StartSwitchRaw_bool"
  Constant/1 -> CoolButtonLatch/2
  CoolButtonLatch/1 -> ?
  Constant1/1 -> ToggleSwitch/2
  ToggleSwitch/1 -> ?
  Constant2/1 -> ToggleSwitch1/2
  ToggleSwitch1/1 -> ?
  Constant3/1 -> ToggleSwitch2/2
  XOR/1 -> ToggleSwitch2/1
  ToggleSwitch2/1 -> ?
  Ground/1 -> OverMeas1/1
  Ground1/1 -> OverMeas3/1
  Ground2/1 -> OverMeas5/1
  Ground3/1 -> OverMeas7/1

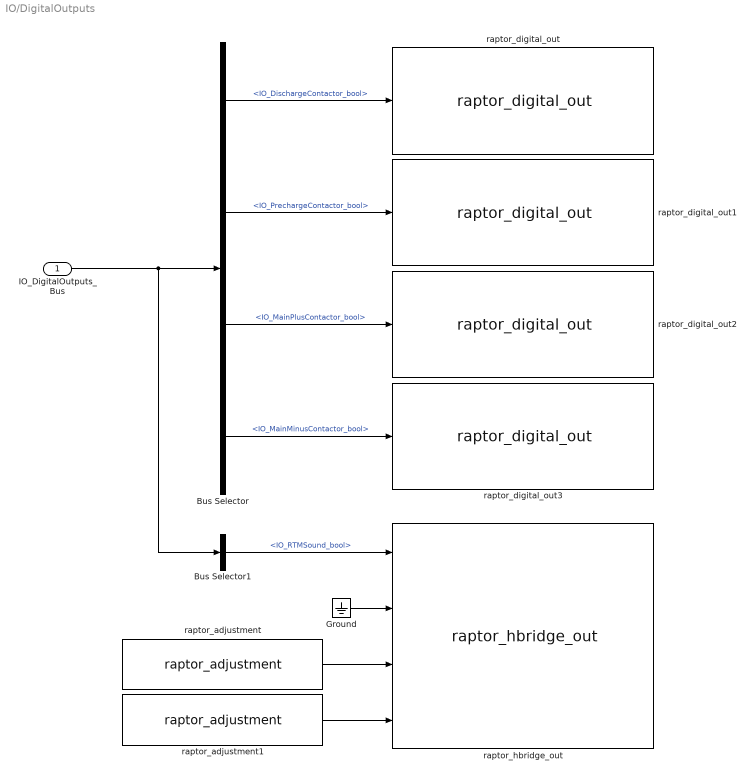
== system IO/DigitalOutputs ==
  IO_DigitalOutputs_Bus : Inport
  Bus Selector : BusSelector  OutputSignals=IO_Contactor_Bus.IO_DischargeContactor_bool,IO_Contactor_Bus.IO_PrechargeContactor_bool,IO_Contactor_Bus.IO_MainPlusContactor_bool,IO_Contactor_Bus.IO_MainMinusContactor_bool
  Bus Selector1 : BusSelector  OutputSignals=IO_RTMSound_bool
  Ground : Ground
  raptor_adjustment : Raptor_lib/Data Storage/raptor_adjustment  paramName='IO_RTMSoundDuty_pct'  nameSource=Parameter  initValue=5000  dataType=int16  storage=Calibration  calDispType=Number  calEnum={'False', 'True'}  calGain=1.0  calOffset=0.0  calMax=inf  calMin=-inf  calFormat='-1'  calUnit=''  calHelp=''  calAccess=1  calFunction=raptor_xcp_function(gcb)  calDispHeaders=off  calColHeaders={'Col1' 'Col2' 'Col3'}  calRowHeaders={'Row1' 'Row2' 'Row3'}
      settings: SourceProductName=Raptor
  raptor_adjustment1 : Raptor_lib/Data Storage/raptor_adjustment  paramName='IO_RTMSoundFreq_Hz'  nameSource=Parameter  initValue=320000  dataType=uint32  storage=Calibration  calDispType=Number  calEnum={'False', 'True'}  calGain=1.0  calOffset=0.0  calMax=inf  calMin=0  calFormat='-1'  calUnit=''  calHelp=''  calAccess=1  calFunction=raptor_xcp_function(gcb)  calDispHeaders=off  calColHeaders={'Col1' 'Col2' 'Col3'}  calRowHeaders={'Row1' 'Row2' 'Row3'}
      settings: SourceProductName=Raptor
  raptor_digital_out : Raptor_lib/Input & Output/raptor_digital_out  resourceValues=OUTPUT1|OUTPUT2|OUTPUT3|OUTPUT4|OUTPUT5|OUTPUT6|OUTPUT7|OUTPUT8|OUTPUT9|OUTPUT10|OUTPUT11|OUTPUT12|OUTPUT21|OUTPUT22|OUTPUT23|OUTPUT24|OUTPUT25|OUTPUT26|OUTPUT27|OUTPUT28|OUTPUT29|OUTPUT30|OUTPUT31|OUTPUT32|OUTPUT33|OUTPUT34|OUTPUT35|OUTPUT36|OUTPUT37|OUTPUT38|OUTPUT39|OUTPUT40|OUTPUT41|OUTPUT42|OUTPUT43|OUTPUT44|OUTPUT45|OUTPUT46|OUTPUT47|OUTPUT48|OUTPUT49|POWER_HOLD|(None)  resource=OUTPUT10  driverTypeValues=Low Side  driverType=Low Side
      settings: SourceProductName=Raptor
  raptor_digital_out1 : Raptor_lib/Input & Output/raptor_digital_out  resourceValues=OUTPUT1|OUTPUT2|OUTPUT3|OUTPUT4|OUTPUT5|OUTPUT6|OUTPUT7|OUTPUT8|OUTPUT9|OUTPUT10|OUTPUT11|OUTPUT12|OUTPUT21|OUTPUT22|OUTPUT23|OUTPUT24|OUTPUT25|OUTPUT26|OUTPUT27|OUTPUT28|OUTPUT29|OUTPUT30|OUTPUT31|OUTPUT32|OUTPUT33|OUTPUT34|OUTPUT35|OUTPUT36|OUTPUT37|OUTPUT38|OUTPUT39|OUTPUT40|OUTPUT41|OUTPUT42|OUTPUT43|OUTPUT44|OUTPUT45|OUTPUT46|OUTPUT47|OUTPUT48|OUTPUT49|POWER_HOLD|(None)  resource=OUTPUT2  driverTypeValues=Low Side  driverType=Low Side
      settings: SourceProductName=Raptor
  raptor_digital_out2 : Raptor_lib/Input & Output/raptor_digital_out  resourceValues=OUTPUT1|OUTPUT2|OUTPUT3|OUTPUT4|OUTPUT5|OUTPUT6|OUTPUT7|OUTPUT8|OUTPUT9|OUTPUT10|OUTPUT11|OUTPUT12|OUTPUT21|OUTPUT22|OUTPUT23|OUTPUT24|OUTPUT25|OUTPUT26|OUTPUT27|OUTPUT28|OUTPUT29|OUTPUT30|OUTPUT31|OUTPUT32|OUTPUT33|OUTPUT34|OUTPUT35|OUTPUT36|OUTPUT37|OUTPUT38|OUTPUT39|OUTPUT40|OUTPUT41|OUTPUT42|OUTPUT43|OUTPUT44|OUTPUT45|OUTPUT46|OUTPUT47|OUTPUT48|OUTPUT49|POWER_HOLD|(None)  resource=OUTPUT9  driverTypeValues=Low Side  driverType=Low Side
      settings: SourceProductName=Raptor
  raptor_digital_out3 : Raptor_lib/Input & Output/raptor_digital_out  resourceValues=OUTPUT1|OUTPUT2|OUTPUT3|OUTPUT4|OUTPUT5|OUTPUT6|OUTPUT7|OUTPUT8|OUTPUT9|OUTPUT10|OUTPUT11|OUTPUT12|OUTPUT21|OUTPUT22|OUTPUT23|OUTPUT24|OUTPUT25|OUTPUT26|OUTPUT27|OUTPUT28|OUTPUT29|OUTPUT30|OUTPUT31|OUTPUT32|OUTPUT33|OUTPUT34|OUTPUT35|OUTPUT36|OUTPUT37|OUTPUT38|OUTPUT39|OUTPUT40|OUTPUT41|OUTPUT42|OUTPUT43|OUTPUT44|OUTPUT45|OUTPUT46|OUTPUT47|OUTPUT48|OUTPUT49|POWER_HOLD|(None)  resource=OUTPUT12  driverTypeValues=Low Side  driverType=Low Side
      settings: SourceProductName=Raptor
  raptor_hbridge_out : Raptor_lib/Input & Output/raptor_hbridge_out  resourceValues=OUTPUT50_51|OUTPUT52_53|OUTPUT54_55|(None)  resource=OUTPUT50_51  outError=0  driverTypeValues=H-Bridge  driverType=H-Bridge
      settings: SourceProductName=Raptor
  wires:
  raptor_adjustment1/1 -> raptor_hbridge_out/4
  raptor_adjustment/1 -> raptor_hbridge_out/3
  Ground/1 -> raptor_hbridge_out/2
  Bus Selector1/1 -> raptor_hbridge_out/1  "<IO_RTMSound_bool>"
  Bus Selector/4 -> raptor_digital_out3/1  "<IO_MainMinusContactor_bool>"
  Bus Selector/3 -> raptor_digital_out2/1  "<IO_MainPlusContactor_bool>"
  Bus Selector/2 -> raptor_digital_out1/1  "<IO_PrechargeContactor_bool>"
  Bus Selector/1 -> raptor_digital_out/1  "<IO_DischargeContactor_bool>"
  IO_DigitalOutputs_Bus/1 -> Bus Selector/1, Bus Selector1/1

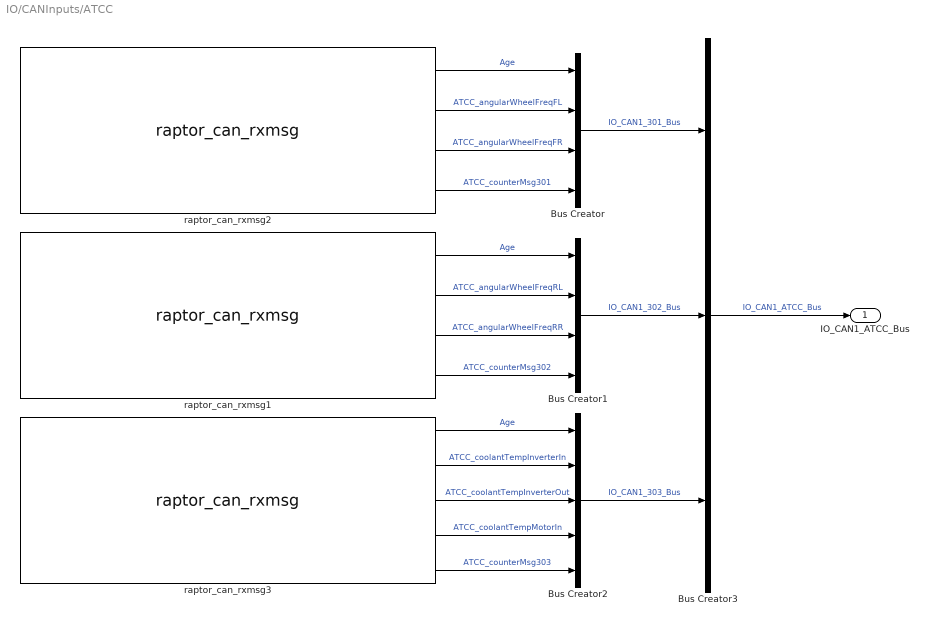
== system IO/CANInputs/ATCC ==
  Bus Creator : BusCreator  Inputs=4
  Bus Creator1 : BusCreator  Inputs=4
  Bus Creator2 : BusCreator  Inputs=5
  Bus Creator3 : BusCreator  Inputs=3
  raptor_can_rxmsg1 : Raptor_lib/CAN/raptor_can_rxmsg  canDefinition=struct('dbcFile', 'raptor_CAN1.dbc','message', 'ATCC_302','comment', '','signals', {{'ATCC_angularWheelFreqRL','ATCC_angularWheelFreqRR','ATCC_counterMsg302'}},'enabled', [ 1 1 1;],'scaled', [ 1 1 1;],'canBus', '''CAN1''','messageID', [ 302;],'idMask', [ 536870911;],'payloadMask', [],'payloadValue', [],'period', [ 0;],'mailbox', '''''','queueSize', [ 1;],'label', [ 1;],'ver', [ 2;],'showID', [ 0;],'showRaw', [ 0;],'showRawMsg', [ 0;],'useStartVals', [ 0;],'extendedId', [ 0;],'showAge', [ 1;],'useSimFunc', [ 0;],'sim_func_name', '''''','fill', [ 0;],'editID', [ 0;],'signalOrder', [ 1;],'signalAscDes', [ 1;],'msgLength', [ 8;])  canBus='CAN1'  mailbox=''  payloadMask=[]  payloadValue=[]  idMask=hex2dec('1FFFFFFF')  queueSize=1  showID=0  label=1  fill=0  id=302  showRaw=0  showAge=1  signalOrder=1  signalInfo={{struct('Name', 'ATCC_counterMsg302','StartBit', [ 0;],'SignalSize', [ 4;],'ByteOrder', 'LittleEndian','ValueType', 'UNSIGNED','Class', 'uint8','Signed', [ 0;],'Factor', [ 1;],'Offset', [ 0;],'Min', [ 0;],'Max', [ 15;],'Units', '','StartVal', [ 0;],'Comment', 'Counter Message 302','Multiplexed', [ 0;],'Multiplexor', [ 0;],'MultiplexMode_Min', [],'MultiplexMode_Max', []),struct('Name', 'ATCC_angularWheelFreqRR','StartBit', [ 32;],'SignalSize', [ 16;],'ByteOrder', 'LittleEndian','ValueType', 'UNSIGNED','Class', 'uint16','Signed', [ 0;],'Factor', [ 1;],'Offset', [ 0;],'Min', [ 0;],'Max', [ 2000;],'Units', 'Hz','StartVal', [ 0;],'Comment', 'RR Angular Wheel Frequency','Multiplexed', [ 0;],'Multiplexor', [ 0;],'MultiplexMode_Min', [],'MultiplexMode_Max', []),struct('Name', 'ATCC_angularWheelFreqRL','StartBit', [ 16;],'SignalSize', [ 16;],'ByteOrder', 'LittleEndian','ValueType', 'UNSIGNED','Class', 'uint16','Signed', [ 0;],'Factor', [ 1;],'Offset', [ 0;],'Min', [ 0;],'Max', [ 2000;],'Units', 'Hz','StartVal', [ 0;],'Comment', 'RL Angular Wheel Frequency','Multiplexed', [ 0;],'Multiplexor', [ 0;],'MultiplexMode_Min', [],'MultiplexMode_Max', [])}}  showRawMsg=0  useSimFunc=0  sim_func_name=''  useStartVals=0  extendedId=0
      settings: SourceProductName=Raptor
  raptor_can_rxmsg2 : Raptor_lib/CAN/raptor_can_rxmsg  canDefinition=struct('dbcFile', 'raptor_CAN1.dbc','message', 'ATCC_301','comment', '','signals', {{'ATCC_angularWheelFreqFL','ATCC_angularWheelFreqFR','ATCC_counterMsg301'}},'enabled', [ 1 1 1;],'scaled', [ 1 1 1;],'canBus', '''CAN1''','messageID', [ 301;],'idMask', [ 536870911;],'payloadMask', [],'payloadValue', [],'period', [ 0;],'mailbox', '''''','queueSize', [ 1;],'label', [ 1;],'ver', [ 2;],'showID', [ 0;],'showRaw', [ 0;],'showRawMsg', [ 0;],'useStartVals', [ 0;],'extendedId', [ 0;],'showAge', [ 1;],'useSimFunc', [ 0;],'sim_func_name', '''''','fill', [ 0;],'editID', [ 0;],'signalOrder', [ 1;],'signalAscDes', [ 1;],'msgLength', [ 8;])  canBus='CAN1'  mailbox=''  payloadMask=[]  payloadValue=[]  idMask=hex2dec('1FFFFFFF')  queueSize=1  showID=0  label=1  fill=0  id=301  showRaw=0  showAge=1  signalOrder=1  signalInfo={{struct('Name', 'ATCC_counterMsg301','StartBit', [ 0;],'SignalSize', [ 4;],'ByteOrder', 'LittleEndian','ValueType', 'UNSIGNED','Class', 'uint8','Signed', [ 0;],'Factor', [ 1;],'Offset', [ 0;],'Min', [ 0;],'Max', [ 15;],'Units', '','StartVal', [ 0;],'Comment', 'Counter Message 301','Multiplexed', [ 0;],'Multiplexor', [ 0;],'MultiplexMode_Min', [],'MultiplexMode_Max', []),struct('Name', 'ATCC_angularWheelFreqFR','StartBit', [ 32;],'SignalSize', [ 16;],'ByteOrder', 'LittleEndian','ValueType', 'UNSIGNED','Class', 'uint16','Signed', [ 0;],'Factor', [ 1;],'Offset', [ 0;],'Min', [ 0;],'Max', [ 2000;],'Units', 'Hz','StartVal', [ 0;],'Comment', 'FR Angular Wheel Frequency','Multiplexed', [ 0;],'Multiplexor', [ 0;],'MultiplexMode_Min', [],'MultiplexMode_Max', []),struct('Name', 'ATCC_angularWheelFreqFL','StartBit', [ 16;],'SignalSize', [ 16;],'ByteOrder', 'LittleEndian','ValueType', 'UNSIGNED','Class', 'uint16','Signed', [ 0;],'Factor', [ 1;],'Offset', [ 0;],'Min', [ 0;],'Max', [ 2000;],'Units', 'Hz','StartVal', [ 0;],'Comment', 'FL Angular Wheel Frequency','Multiplexed', [ 0;],'Multiplexor', [ 0;],'MultiplexMode_Min', [],'MultiplexMode_Max', [])}}  showRawMsg=0  useSimFunc=0  sim_func_name=''  useStartVals=0  extendedId=0
      settings: SourceProductName=Raptor
  raptor_can_rxmsg3 : Raptor_lib/CAN/raptor_can_rxmsg  canDefinition=struct('dbcFile', 'raptor_CAN1.dbc','message', 'ATCC_303','comment', '','signals', {{'ATCC_coolantTempInverterIn','ATCC_coolantTempInverterOut','ATCC_coolantTempMotorIn','ATCC_counterMsg303'}},'enabled', [ 1 1 1 1;],'scaled', [ 1 1 1 1;],'canBus', '''CAN1''','messageID', [ 303;],'idMask', [ 536870911;],'payloadMask', [],'payloadValue', [],'period', [ 0;],'mailbox', '''''','queueSize', [ 1;],'label', [ 1;],'ver', [ 2;],'showID', [ 0;],'showRaw', [ 0;],'showRawMsg', [ 0;],'useStartVals', [ 0;],'extendedId', [ 0;],'showAge', [ 1;],'useSimFunc', [ 0;],'sim_func_name', '''''','fill', [ 0;],'editID', [ 0;],'signalOrder', [ 1;],'signalAscDes', [ 1;],'msgLength', [ 8;])  canBus='CAN1'  mailbox=''  payloadMask=[]  payloadValue=[]  idMask=hex2dec('1FFFFFFF')  queueSize=1  showID=0  label=1  fill=0  id=303  showRaw=0  showAge=1  signalOrder=1  signalInfo={{struct('Name', 'ATCC_counterMsg303','StartBit', [ 0;],'SignalSize', [ 4;],'ByteOrder', 'LittleEndian','ValueType', 'UNSIGNED','Class', 'uint8','Signed', [ 0;],'Factor', [ 1;],'Offset', [ 0;],'Min', [ 0;],'Max', [ 15;],'Units', '','StartVal', [ 0;],'Comment', 'Counter Message 303','Multiplexed', [ 0;],'Multiplexor', [ 0;],'MultiplexMode_Min', [],'MultiplexMode_Max', []),struct('Name', 'ATCC_coolantTempMotorIn','StartBit', [ 16;],'SignalSize', [ 16;],'ByteOrder', 'LittleEndian','ValueType', 'SIGNED','Class', 'int16','Signed', [ 1;],'Factor', [ 0.1;],'Offset', [ 0;],'Min', [ 0;],'Max', [ 120;],'Units', 'degC','StartVal', [ 0;],'Comment', 'Motor In Coolant Temperature','Multiplexed', [ 0;],'Multiplexor', [ 0;],'MultiplexMode_Min', [],'MultiplexMode_Max', []),struct('Name', 'ATCC_coolantTempInverterOut','StartBit', [ 48;],'SignalSize', [ 16;],'ByteOrder', 'LittleEndian','ValueType', 'SIGNED','Class', 'int16','Signed', [ 1;],'Factor', [ 0.1;],'Offset', [ 0;],'Min', [ 0;],'Max', [ 120;],'Units', 'degC','StartVal', [ 0;],'Comment', 'Inverter Out Coolant Temperature','Multiplexed', [ 0;],'Multiplexor', [ 0;],'MultiplexMode_Min', [],'MultiplexMode_Max', []),struct('Name', 'ATCC_coolantTempInverterIn','StartBit', [ 32;],'SignalSize', [ 16;],'ByteOrder', 'LittleEndian','ValueType', 'SIGNED','Class', 'int16','Signed', [ 1;],'Factor', [ 0.1;],'Offset', [ 0;],'Min', [ 0;],'Max', [ 120;],'Units', 'degC','StartVal', [ 0;],'Comment', 'Inverter In Coolant Temperature','Multiplexed', [ 0;],'Multiplexor', [ 0;],'MultiplexMode_Min', [],'MultiplexMode_Max', [])}}  showRawMsg=0  useSimFunc=0  sim_func_name=''  useStartVals=0  extendedId=0
      settings: SourceProductName=Raptor
  IO_CAN1_ATCC_Bus : Outport
  wires:
  Bus Creator3/1 -> IO_CAN1_ATCC_Bus/1  "IO_CAN1_ATCC_Bus"
  Bus Creator2/1 -> Bus Creator3/3  "IO_CAN1_303_Bus"
  Bus Creator/1 -> Bus Creator3/1  "IO_CAN1_301_Bus"
  Bus Creator1/1 -> Bus Creator3/2  "IO_CAN1_302_Bus"
  raptor_can_rxmsg3/5 -> Bus Creator2/5  "ATCC_counterMsg303"
  raptor_can_rxmsg3/4 -> Bus Creator2/4  "ATCC_coolantTempMotorIn"
  raptor_can_rxmsg3/3 -> Bus Creator2/3  "ATCC_coolantTempInverterOut"
  raptor_can_rxmsg3/2 -> Bus Creator2/2  "ATCC_coolantTempInverterIn"
  raptor_can_rxmsg3/1 -> Bus Creator2/1  "Age"
  raptor_can_rxmsg1/4 -> Bus Creator1/4  "ATCC_counterMsg302"
  raptor_can_rxmsg1/3 -> Bus Creator1/3  "ATCC_angularWheelFreqRR"
  raptor_can_rxmsg1/2 -> Bus Creator1/2  "ATCC_angularWheelFreqRL"
  raptor_can_rxmsg1/1 -> Bus Creator1/1  "Age"
  raptor_can_rxmsg2/4 -> Bus Creator/4  "ATCC_counterMsg301"
  raptor_can_rxmsg2/3 -> Bus Creator/3  "ATCC_angularWheelFreqFR"
  raptor_can_rxmsg2/2 -> Bus Creator/2  "ATCC_angularWheelFreqFL"
  raptor_can_rxmsg2/1 -> Bus Creator/1  "Age"
